simulink library "PowerFlowLib2013aslx"  (R2013a)
settings: Solver=ode45  StartTime=0.0  StopTime=10.0  RelTol=1e-3
undefined symbols (not defined in the file or in its folder): AirProp, C, F1, Fanmap, Fld1, Fld2, fueltankdata, HydProp, HydraulicLoad, IBFD_exc, L, LoadFluidProps, magnitude, MSSN, n_alghts, PumpProp, pwr_alghts, R_fd_exc, Rcore, Ts, VBFD_exc
libraries: PowerFlowLib x32, simulink x14, powerlib_extras x2, dspstat3 x2
(part 1 of 11)
settings Model: Creator=mwillms4  LastModifiedBy=srikanthan

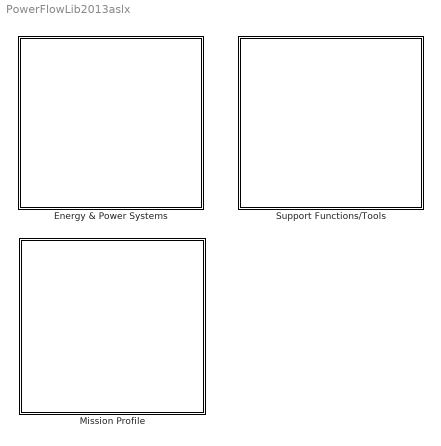
== system PowerFlowLib2013aslx ==
  Energy & Power Systems : Subsystem
      mask Display: color('white')
  Mission Profile : Subsystem
      mask Display: color('white')
  Support Functions/Tools : Subsystem
      mask Display: color('white')

== system PowerFlowLib2013aslx/Energy & Power Systems ==
  Additional Systems : Subsystem
  Electrical : Subsystem
  Hydraulic : Subsystem
  Thermal : Subsystem

== system PowerFlowLib2013aslx/Mission Profile ==
  Mission Profile : Subsystem  InitFcn=|  mask(MISSION PROFILE SELECT){mssn_prof=MSSN, del_P=0, del_T=0, del_rho=0, pres_msl=101.3, temp_msl=15, dens_msl=1.229}
      | h      = get_param(gcb,'handle');   % Get block handle
      | blk    = gcb; 
      | hblock = get(h);     % Parse out handles structure 
      | 
      | if ((exist(hblock.mssn_prof) == 0) && (strcmp('blank',hblock.mssn_prof) ~= 1))
      |     open_system(gcb)
      |     msgbox(['Aborting simulation due to invalid mission profile selected. ', hblock.mssn_prof,' does not exist in workspace.']);
      |     set_param(bdroot,'SimulationCommand','stop')
      | end
      | 
      | 
      | 
      | clear h blk hblock
      mask prompts: mssn_prof "Mission Profile Variable (from workspace)"; del_P "Pres. deviation from standard atmospheric conditions [kPa]"; del_T "Temp. deviation from standard atmospheric conditions [°C]"; del_rho "Density Deviation from standard"; pres_msl "MSL Pressure [kPa]"; temp_msl "MSL Temperature [°C]"; dens_msl "MSL Density [kg/m³]"
      mask help:
      | Select the MATLAB workspace variable that contains mission specifications. This variable should be created with the automated code included with the PowerFlow toolset.
      |
      | Also specify deviations from standard atmospheric conditions.
